simulink model "model_sterowania"  (R2023a)
settings: Solver=ode45  StartTime=0.0  StopTime=sim_time  FixedStep=0.001  RelTol=1e-3  EnableMultiTasking=on
values from neighbouring files (symbols this model uses):
  a = 27.62    [parametry.m]
  b = -304.84    [parametry.m]
  c = 112.75    [parametry.m]
  d = -2.74    [parametry.m]
  g = 9.81    [parametry.m]
  m = 0.058    [parametry.m]
  R = 1    [linearize_model.m]    (also in parametry.m = 4.38)
  u_max = 12.28    [parametry.m]
settings Model: Creator=Student  LastModifiedBy=HP
settings SolverCC: AlgebraicLoopSolver=TrustRegion
settings DataIOCC: SaveFormat=Array  ReturnWorkspaceOutputs=off
settings OptimizationCC: LifeSpan=inf
settings DebuggingCC: UnconnectedInputMsg=warning  UnconnectedOutputMsg=warning  UnconnectedLineMsg=warning  SFUnexpectedBacktrackingDiag=warning  SFNoUnconditionalDefaultTransitionDiag=warning  SFExecutionAtInitializationDiag=none  ArithmeticOperatorsInVariantConditions=warning
settings HardwareCC: ProdBitPerPointer=32  ProdBitPerSizeT=32  ProdBitPerPtrDiffT=32  ProdLargestAtomicFloat=None  ProdIntDivRoundTo=Undefined  ProdEndianess=Unspecified  ProdWordSize=32  ProdHWDeviceType=32-bit Generic
settings ModelReferenceCC: PropagateSignalLabelsOutOfModel=off
settings SFSimCC: SimUseLocalCustomCode=off  CustomCodeUndefinedFunction=UseInterfaceOnly
settings RTWCC: RTWUseLocalCustomCode=off
settings CodeAppCC: StateflowObjectComments=on
settings GRTTargetCC: TargetLangStandard=C89/C90 (ANSI)
settings ConfigComp: CovMetricSettings=dw  CovSaveCumulativeToWorkspaceVar=on  CovSaveSingleToWorkspaceVar=on  CovExternalEMLEnable=off

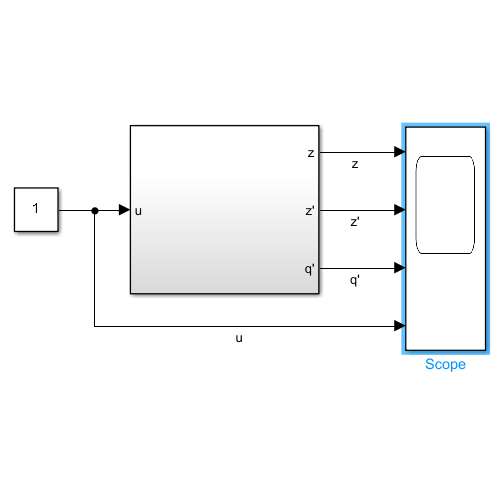
[thumbnail: Simulink's stored preview of the top-level diagram]
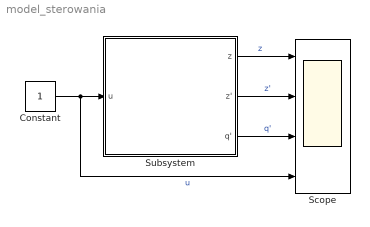
== system model_sterowania ==
  Constant : Constant
  Scope : Scope  NumInputPorts=4
  Subsystem : Subsystem
  wires:
  Constant/1 -> Scope/4, Subsystem/1(u)  "u"
  Subsystem/3(q') -> Scope/3  "q'"
  Subsystem/2(z') -> Scope/2  "z'"
  Subsystem/1(z) -> Scope/1  "z"

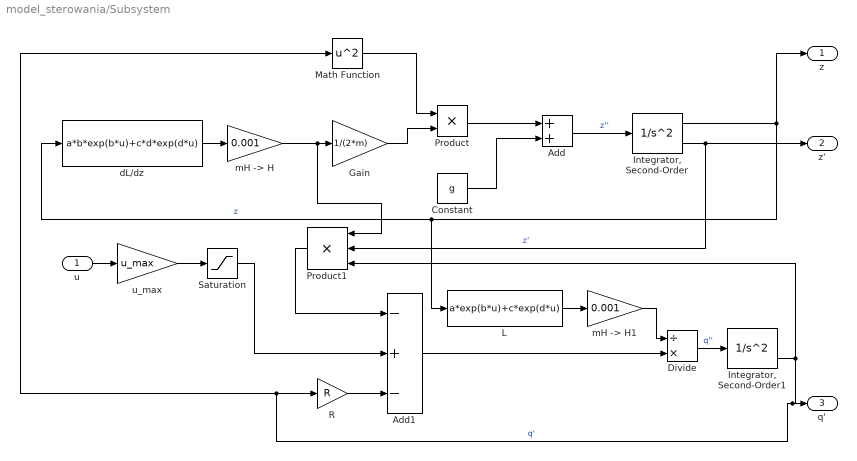
== system model_sterowania/Subsystem ==
  u : Inport
  Add : Sum
  Add1 : Sum  Inputs=-+-
  Constant : Constant  Value=g
  Divide : Product  Inputs=/*
  Gain : Gain  Gain=1/(2*m)
  "Integrator, Second-Order" : SecondOrderIntegrator  ICX=x0  LimitX=on  UpperLimitX=0.025  LowerLimitX=0
  "Integrator, Second-Order1" : SecondOrderIntegrator  ICX=q0
  L : Fcn  Expr=a*exp(b*u)+c*exp(d*u)
  Math Function : Math  Operator=square  SignedPower=on
  Product : Product
  Product1 : Product  Inputs=3
  R : Gain  Gain=R
  Saturation : Saturate  UpperLimit=12  LowerLimit=0
  dL/dz : Fcn  Expr=a*b*exp(b*u)+c*d*exp(d*u)
  "mH -> H" : Gain  Gain=0.001
  "mH -> H1" : Gain  Gain=0.001
  u_max : Gain  Gain=u_max
  z : Outport
  z' : Outport  Port=2
  q' : Outport  Port=3
  wires:
  Math Function/1 -> Product/1
  Constant/1 -> Add/2
  Product/1 -> Add/1
  Gain/1 -> Product/2
  "Integrator, Second-Order"/2 -> Product1/2, z'/1  "z'"
  R/1 -> Add1/3
  Add/1 -> "Integrator, Second-Order"/1  "z''"
  Saturation/1 -> Add1/2
  u/1 -> u_max/1
  u_max/1 -> Saturation/1
  "Integrator, Second-Order1"/2 -> Product1/3, R/1, Math Function/1, q'/1  "q'"
  Divide/1 -> "Integrator, Second-Order1"/1  "q''"
  "Integrator, Second-Order"/1 -> dL/dz/1, L/1, z/1  "z"
  Product1/1 -> Add1/1
  dL/dz/1 -> "mH -> H"/1
  Add1/1 -> Divide/2
  "mH -> H"/1 -> Product1/1, Gain/1
  L/1 -> "mH -> H1"/1
  "mH -> H1"/1 -> Divide/1
